simulink model "svpwm_inv_Motor_new_sent_split4"  (R2023a)
settings: Solver=daessc  StartTime=0.0  StopTime=0.62  MaxStep=2.5e-7  RelTol=1e-3
undefined symbols (not defined in the file): DiscIntNeverNeededParam
libraries: nesl_utility x37, fl_lib x34, ee_lib x21, spsMeanLib x7, simulink x6, mcbcontrolslib x4, slpidlib x4, sdl_lib x2, simulink_extras x1
(part 1 of 2)
settings Model: SimulationMode=rapid-accelerator  Creator=alexey  LastModifiedBy=alexey
settings SolverCC: ZeroCrossAlgorithm=Adaptive
settings OptimizationCC: ReuseModelBlockBuffer=off
settings DebuggingCC: IgnoredZcDiagnostic=none
settings GRTTargetCC: RTWCAPISignals=on  RTWCAPIParams=on

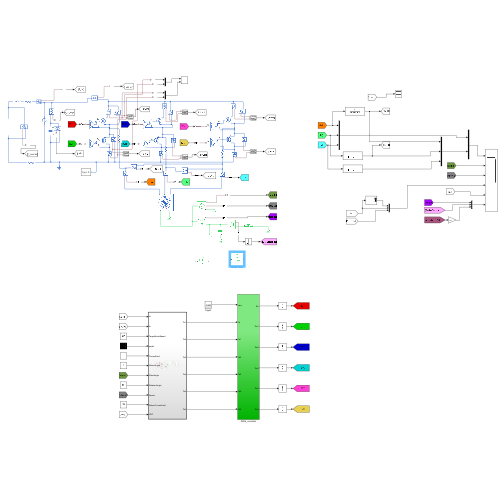
[thumbnail: Simulink's stored preview of the top-level diagram]
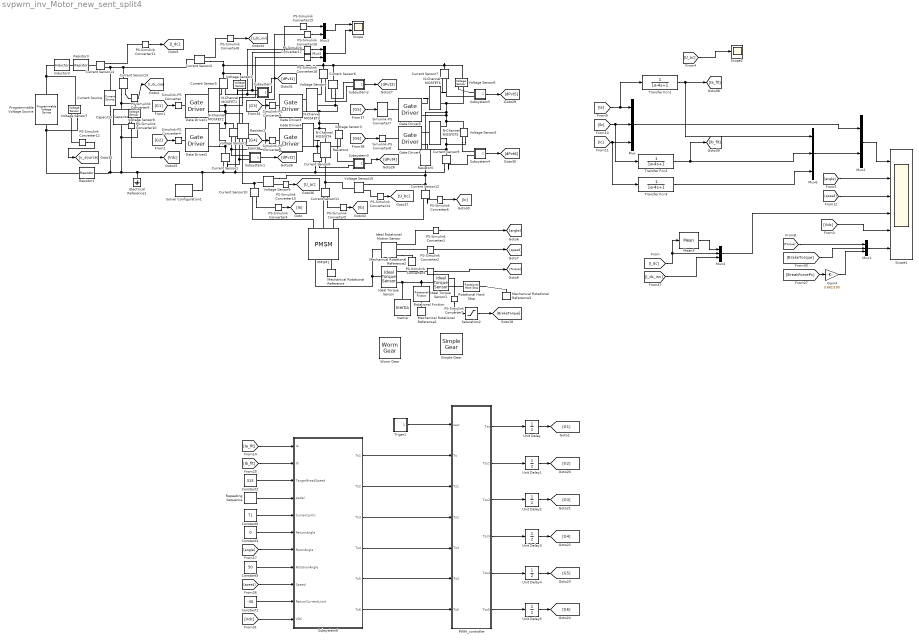
== system svpwm_inv_Motor_new_sent_split4 ==
  Capacitor : fl_lib/Electrical/Electrical Elements/Capacitor  c=270 uF  r=2 mOhm  g=0 1/Ohm  i_specify=off  i_priority=None  i=0 A  i_nominal_specify=off  i_nominal_unit=A  i_nominal_value=1  v_specify=on  v_priority=None  v=0 V  v_nominal_specify=off  v_nominal_unit=V  v_nominal_value=1  vc_specify=off  vc_priority=High  vc=0 V  vc_nominal_specify=off  vc_nominal_unit=V  vc_nominal_value=1
  Constant1 : Constant  Value=-30
  Constant2 : Constant  Value=315
  Constant4 : Constant  Value=0
  Constant5 : Constant  Value=50
  Constant6 : Constant  Value=71
  Current Sensor{1..2,5..14} (12 alike) : fl_lib/Electrical/Electrical Sensors/Current Sensor
  Current Source : ee_lib/Sources/Current Source  dc_current=0.25 A  ac_current=0 A  ac_shift=0 rad  ac_frequency=60 Hz  noise_mode=ee.enum.sources.noise.Disabled  PSD=0 A^2/Hz  sample_time=1e-3 s  repeatability=ee.enum.sources.repeatability.NotRepeatable  user_seed=0  auto_seed=3499211588  i_specify=off  i_priority=None  i=0 A  i_nominal_specify=off  i_nominal_unit=A  i_nominal_value=1  v_specify=off  v_priority=None  v=0 V  v_nominal_specify=off  v_nominal_unit=V  v_nominal_value=1
  Electrical Reference1 : fl_lib/Electrical/Electrical Elements/Electrical Reference
  Gain4 : Gain  Gain=3.682/100
  Gate Driver{1..6} (6 alike) : ee_lib/Semiconductors & Converters/Gate Driver  uHighValue=0.7  uLowValue=0.3  vHigh=12 V  vLow=0 V  tHigh=50 ns  tLow=50 ns  parameterization=1  rHigh=2 Ohm  rLow=2 Ohm  tRise=20 ns  tFall=20 ns  cLoad=10 nF  enable_faults=0  t_fault=1 s  fault_type=1  ZonTime_specify=off  ZonTime_priority=None  ZonTime=0 s  ZoffTime_specify=off  ZoffTime_priority=None  ZoffTime=0 s  uHigh=2.0 V  uLow=0.8 V
      settings: InternalSimscapePortConfiguration="{\"Bottom\":[],\"Left\":[{\"id\":\"u\",\"label\":\"u\",\"type\":\"input\"}],\"Right\":[{\"id\":\"G\",\"label\":\"G\",\"type\":\"foundation.electrical.electrical\"},{\"id\":\"S\",\"label\":\"S\",\"type\":\"foundation.electrical.electrical\"}],\"Top\":[]}"
  Ideal Rotational Motion Sensor : fl_lib/Mechanical/Mechanical Sensors/Ideal Rotational Motion Sensor  reference=foundation.enum.MeasurementReference.difference  acceleration_port=false  velocity_port=true  position_port=true  wrap_angle=false  offset=0 rad
  Ideal Torque Sensor : fl_lib/Mechanical/Mechanical Sensors/Ideal Torque Sensor
  Ideal Torque Sensor1 : fl_lib/Mechanical/Mechanical Sensors/Ideal Torque Sensor
  Inductor3 : ee_lib/Passive/Inductor  l=1 uH  enable_L_tol=0  L_tol=20  tol_distribution=1  nSigma=4  r=0 Ohm  g=1e-9 1/Ohm  enable_operating_limits=0  operating_limit_action=2  max_working_current=1 A  power_rating=1 W  enable_faults=ee.enum.enable.no  fault_action=simscape.enum.assert.action.none  lambdaPercent=50  k_faulted=0.9999  turnsShort=0  openCct=0  groundShort=0  groundShortG=0 1/Ohm  tau_fault=1e-3 s  fault_trigger=ee.enum.faults.faultTrigger.temporal  t_fault=1 s  max_permissible_voltage=100 V  n_fail_on_voltage=1  max_permissible_current=1 A  t_fail_on_current=1 s  i_L_specify=on  i_L_priority=High  i_L=0 A  i_L_nominal_specify=off  i_L_nominal_unit=A  i_L_nominal_value=1
  Inertia : fl_lib/Mechanical/Rotational Elements/Inertia  inertia=3e-5 kg*m^2  num_ports=foundation.enum.numPorts2.one  w_specify=off  w_priority=High  w=0 rad/s  w_nominal_specify=off  w_nominal_unit=rad/s  w_nominal_value=1  t_specify=off  t_priority=None  t=0 N*m  t_nominal_specify=off  t_nominal_unit=N*m  t_nominal_value=1
  Mean3 : spsMeanLib/Mean  Freq=10000  Vinit=0  Ts=0
  Mechanical Rotational Reference{,1..3} (4 alike) : fl_lib/Mechanical/Rotational Elements/Mechanical Rotational Reference
  Mux{,1,4,6} (4 alike) : Mux  Inputs=3
  Mux2 : Mux  Inputs=2
  Mux3 : Mux  Inputs=2
  Mux5 : Mux  Inputs=2
  N-Channel MOSFET{1..6} (6 alike) : ee_lib/Semiconductors & Converters/N-Channel MOSFET  paramTerminal=ee.enum.mosfet.numberOfTerminals.three  parameterization=ee.enum.mosfet.parameterization.datasheet  Beta=5.0 A/V^2  Rds=0.85 mOhm  Id=100 A  Vgs=10 V  Vth=2.6 V  Vth0=1.7 V  lam=0 1/V  gamma_vth=0.5 V^(1/2)  phib=0.5 V  Vth1=1.9071 V  Vbs1=-1 V  Vth2=2.066 V  Vbs2=-2 V  Tmeas=25 degC  Vgs_vec=[-.5, 2, 3, 4, 5] V  Vds_vec=[0, 2, 4, 8, 12, 16, 20] V  Vbs_vec=[0, -4, -6, -12] V  T_vec=[25, 125] degC  Vth_vec=[.4, 1.2, 1.4, 1.45] V  Vth_mat=[.4, .35; 1.2, 1.15; 1.4, 1.35; 1.45, 1.4] V  Ids_mat=[0, 0, 0, 0, 0, 0, 0; 0, .003, .0038, .0043, .0046, .0048, .0049; 0, .0055, .008, .009, .0095, .01, .0101; 0, .0115, .016, .018, .019, .0195, .02; 0, .0152, .0225, .0265, .028, .0295, .03] A  Ids_mat0=[0, 0, 0, 0, 0, 0, 0; 0, .003, .0038, .0043, .0046, .0048, .0049; 0, .0055, .008, .009, .0095, .01, .0101; 0, .0115, .016, .018, .019, .0195, .02; 0, .0152, .0225, .0265, .028, .0295, .03] A  Ids_mat_3D=zeros(5, 7, 2) A  Ids_mat_3D0=zeros(5, 7, 2) A  IV_table_symmetry=ee.enum.mosfet.symmetricNIV.no  RS=0.0001 Ohm  RD=0.0001 Ohm  RB=0.001 Ohm  C_param=ee.enum.mosfet.capacitanceParam.tabulatedciss  C_GS=270 pF  C_GD=80 pF  C_GB=0 pF  C_DS=0 pF  C_iss=350 pF  C_rss=80 pF  C_oss=0 pF  C_iss_vec=[19000, 17000, 16500, 16500, 16000, 16000, 16000, 16000, 16000] pF  C_rss_vec=[3100, 1700, 750, 280, 110, 90, 80, 80, 80] pF  C_oss_vec=[16000, 11000, 8000, 6500, 3000, 2800, 2650, 2600, 2400] pF  C_GS_vec=[270, 300, 290, 280, 295, 255] pF  C_GD_vec=[450, 400, 300, 190, 95, 55] pF  C_GB_vec=[270, 300, 290, 280, 295, 255] pF  C_Vgs_vec=0 V  C_DS_vec=[450, 410, 390, 230, 175, 115] pF  C_Vds_vec=[.1, 4, 12, 20, 28, 36, 44, 52, 60] V  V_GS_for_cap_data=0 V  charge_linearity_param=ee.enum.mosfet.cgdLinearity.constant  C_OX=200 pF  V_C_OX=-0.5 V  charge_linearity_param_vgb=ee.enum.mosfet.cgbLinearity.instantly  charge_linearity_param_with_vgb=ee.enum.mosfet.cgbLinearityWithSeparateCgb.instantly  Di_param=ee.enum.mosfet.diodeParam.tabulated  IsDiode=1e-12 A  Vbi=0.18 V  n=1  Cj0Diode=9000 pF  TT=50e-9 s  Tmeas_dio=25 degC  TableTypeNoT=ee.enum.mosfet.tableType.IfMat  TableType=ee.enum.diode.tableType.IfMat  IfVec=[1e-3, 1, 10, 100, 400, 1000] A  IfMat=[.07, .12, .19, 1.75, 4.24, 7.32, 11.2; .16, .3, .72, 2.14, 4.02, 6.35, 9.12] A  VfVecV=[.9, 1.15, 1.25, 1.5, 1.75, 2.17, 2.6, 2.85] V  VfMatV=[.9, 1.15, 1.25, 1.5, 1.75, 2.17, 2.6, 2.85; .58, .68, .75, 1.1, 1.38, 1.77, 2.27, 2.7] V  TjVec=[25, 125] degC  VfVec=[0.68, 0.69, 0.72, 0.82, 0.9, 1.1] V  IfVecV=[.1, .2, .5, 1, 2, 4, 7, 10] A  prmDatasheet=ee.enum.temperatureParameterization.none  prmEquCoeff=ee.enum.temperatureParameterization.none  dVth_dT=-6 mV/K  dVth0_dT=-6 mV/K  Rds_T2=0.037 Ohm  BEXDatasheet=-1.5  BEXEquCoeff=-1.5  etaisDatasheet=3  etaisEquCoeff=3  Tmeas2=125 degC  etaisTabulated=3  TdeviceDatasheet=25 degC  TdeviceEquCoeff=25 degC  TdeviceTabulated=25 degC  enable_faults=simscape.enum.onoff.off  fault_trigger=ee.enum.faults.faultTrigger.temporal  t_fault=inf s  max_permissible_Vgs=inf V  max_permissible_Vds=inf V  max_permissible_Vdb=inf V  max_permissible_Ids=inf A  t_fail_on_Ids=1 s  max_permissible_Idiode=inf A  t_fail_on_Idiode=1 s  max_permissible_dVdt=inf V/s  tau_fault=1e-3 s  fault_types=ee.enum.mosfet.faults.open  fault_types_4T=ee.enum.mosfet.faultsFourTerminals.open  RG_open=1e6 Ohm  RD_open=1000 Ohm  RS_open=1000 Ohm  RB_open=1000 Ohm  GDS_short=1000 1/Ohm  GDB_short=1000 1/Ohm  GSB_short=1000 1/Ohm  location_GOS=0  G_GOS=1000 1/Ohm  D_GOS=ee.enum.include.no  Is_GOS=0 A  Vbi_GOS=0.6 V  n_GOS=1  Cj0_GOS=0 pF  TT_GOS=50e-9 s  Beta_scale=100  dVth_faulted=0 V  lam_faulted=0 1/V  gamma_scale=100  dPhib_faulted=0 V  Vgs_vec_faulted=[-.5, 2, 3, 4, 5] V  Vds_vec_faulted=[0, 2, 4, 8, 12, 16, 20] V  Vbs_vec_faulted=[0, -4, -6, -12] V  Vth_vec_faulted=[.4, 1.2, 1.4, 1.45] V  Vth_mat_faulted=[.4, .35; 1.2, 1.15; 1.4, 1.35; 1.45, 1.4] V  Ids_mat_faulted=[0, 0, 0, 0, 0, 0, 0; 0, .003, .0038, .0043, .0046, .0048, .0049; 0, .0055, .008, .009, .0095, .01, .0101; 0, .0115, .016, .018, .019, .0195, .02; 0, .0152, .0225, .0265, .028, .0295, .03] A  Ids_mat0_faulted=[0, 0, 0, 0, 0, 0, 0; 0, .003, .0038, .0043, .0046, .0048, .0049; 0, .0055, .008, .009, .0095, .01, .0101; 0, .0115, .016, .018, .019, .0195, .02; 0, .0152, .0225, .0265, .028, .0295, .03] A  Ids_mat_3D_faulted=zeros(5, 7, 2) A  Ids_mat_3D0_faulted=zeros(5, 7, 2) A  RS_faulted=0.0001 Ohm  RD_faulted=0.01 Ohm  RB_faulted=0.001 Ohm  IsDiode_faulted=0 A  Vbi_faulted=0.6 V  n_faulted=1  Cj0Diode_scale=100  TT_faulted=50e-9 s  IfVec_faulted=[.07, .12, .19, 1.75, 4.24, 7.32, 11.2] A  IfMat_faulted=[.07, .12, .19, 1.75, 4.24, 7.32, 11.2; .16, .3, .72, 2.14, 4.02, 6.35, 9.12] A  VfVecV_faulted=[.9, 1.15, 1.25, 1.5, 1.75, 2.17, 2.6, 2.85] V  VfMatV_faulted=[.9, 1.15, 1.25, 1.5, 1.75, 2.17, 2.6, 2.85; .58, .68, .75, 1.1, 1.38, 1.77, 2.27, 2.7] V  VfVec_faulted=[.5, .7, .9, 1.3, 1.7, 2.1, 2.5] V  IfVecV_faulted=[.1, .2, .5, 1, 2, 4, 7, 10] A  C_GS_scale=100  C_GD_scale=100  C_GB_scale=100  C_DS_scale=100  C_OX_scale=100  V_C_OX_faulted=-0.5 V  C_iss_vec_faulted=[720, 700, 590, 470, 390, 310] pF  C_rss_vec_faulted=[450, 400, 300, 190, 95, 55] pF  C_oss_vec_faulted=[900, 810, 690, 420, 270, 170] pF  C_GS_vec_faulted=[270, 300, 290, 280, 295, 255] pF  C_GD_vec_faulted=[450, 400, 300, 190, 95, 55] pF  C_GB_vec_faulted=[270, 300, 290, 280, 295, 255] pF  C_Vgs_vec_faulted=0 V  C_DS_vec_faulted=[450, 410, 390, 230, 175, 115] pF  C_Vds_vec_faulted=[.1, .3, 1, 3, 10, 30] V  V_GS_for_cap_data_faulted=0 V  i_g_specify=off  i_g_priority=None  i_g=0 A  i_g_nominal_specify=off  i_g_nominal_unit=A  i_g_nominal_value=1  i_d_specify=on  i_d_priority=High  i_d=100 A  i_d_nominal_specify=off  i_d_nominal_unit=A  i_d_nominal_value=1  i_b_specify=off  i_b_priority=None  i_b=0 A  i_b_nominal_specify=off  i_b_nominal_unit=A  i_b_nominal_value=1  voltage_gs_specify=on  voltage_gs_priority=High  voltage_gs=0 V  voltage_gs_nominal_specify=off  voltage_gs_nominal_unit=V  voltage_gs_nominal_value=1  voltage_ds_specify=off  voltage_ds_priority=High  voltage_ds=12 V  voltage_ds_nominal_specify=off  voltage_ds_nominal_unit=V  voltage_ds_nominal_value=1  voltage_bs_specify=off  voltage_bs_priority=None  voltage_bs=0 V  voltage_bs_nominal_specify=off  voltage_bs_nominal_unit=V  voltage_bs_nominal_value=1  v_Cgs_specify=on  v_Cgs_priority=High  v_Cgs=0 V  v_Cgs_nominal_specify=off  v_Cgs_nominal_unit=V  v_Cgs_nominal_value=1  v_Cds_specify=on  v_Cds_priority=High  v_Cds=0 V  v_Cds_nominal_specify=off  v_Cds_nominal_unit=V  v_Cds_nominal_value=1  v_Cbs_specify=off  v_Cbs_priority=High  v_Cbs=0 V  v_Cbs_nominal_specify=off  v_Cbs_nominal_unit=V  v_Cbs_nominal_value=1  thermal_network_parameterization=ee.enum.thermalNetworkTopology.junctionCase  Rth=[0, 10] K/W  Rth_Cauer=[1, 3, 10] K/W  Rth_Foster=[4, 6] K/W  thermal_mass_parameterization=ee.enum.thermalNetwork.timeconstant  thermal_mass=[0, 1] J/K  thermal_mass_Cauer=[.1, .3, 1] J/K  thermal_mass_Foster=[1.5, 3] J/K  thermal_time_constant=[0, 10] s  thermal_time_constant_Cauer=[1, 3, 10] s  thermal_time_constant_Foster=[6, 18] s  thermal_mass_initial_temperatures=[25, 25] degC  thermal_mass_initial_temperatures_Cauer=[25, 25, 25] degC  Tvec_initial_Foster=[25, 25, 25, 25] degC  max_permissible_temperature=inf K  t_fail_on_temperature=1 s  betaref=18 A/V^2  Vfbref=-1.1 V  gamma=3.5 V^(1/2)  phib2ref=1 V  thesatref=0.4 1/V  alpha=0  Vp=5e-2 V  thesrref=0 1/V  m=8  Tref=25 degC  Rsref=2e-3 Ohm  Rdref=0.17 Ohm  Rgref=8.4 Ohm  Rbref=2e-3 Ohm  Cox=1500 pF  Cgso=100 pF  Cgdo=14 pF  Isref=5.2e-13 A  Cj0=480 pF  Tprm=1  etabet=1.3  Stvfb=5e-4 V/K  Stphib=-8.5e-4 V/K  etasat=1.04  etasr=0.65  etar=0.95  etais=3  Tsim=25 degC  Ig_specify=off  Ig_priority=None  Ig=0 A  Ig_nominal_specify=off  Ig_nominal_unit=A  Ig_nominal_value=1  Ids_specify=off  Ids_priority=None  Ids=0 A  Ids_nominal_specify=off  Ids_nominal_unit=A  Ids_nominal_value=1  Ib_specify=off  Ib_priority=None  Ib=0 A  Ib_nominal_specify=off  Ib_nominal_unit=A  Ib_nominal_value=1  V_gs_specify=off  V_gs_priority=None  V_gs=0 V  V_gs_nominal_specify=off  V_gs_nominal_unit=V  V_gs_nominal_value=1  V_ds_specify=off  V_ds_priority=None  V_ds=0 V  V_ds_nominal_specify=off  V_ds_nominal_unit=V  V_ds_nominal_value=1  V_bs_specify=off  V_bs_priority=None  V_bs=0 V  V_bs_nominal_specify=off  V_bs_nominal_unit=V  V_bs_nominal_value=1  QGoverCox_specify=off  QGoverCox_priority=None  QGoverCox=0 V  QGoverCox_nominal_specify=off  QGoverCox_nominal_unit=V  QGoverCox_nominal_value=1  QDoverCox_specify=off  QDoverCox_priority=None  QDoverCox=0 V  QDoverCox_nominal_specify=off  QDoverCox_nominal_unit=V  QDoverCox_nominal_value=1  QBoverCox_specify=off  QBoverCox_priority=None  QBoverCox=0 V  QBoverCox_nominal_specify=off  QBoverCox_nominal_unit=V  QBoverCox_nominal_value=1  T0=[25, 25] degC  T0_Cauer=[25, 25, 25] degC
  PMSM1 : ee_lib/Electromechanical/Permanent Magnet/PMSM  port_option=ee.enum.threePhasePort.expanded  winding_type=ee.enum.statorconnection.delta  machine_param=ee.enum.pmsm.parameterization.constant  nPolePairs=4  pmflux_param=ee.enum.pmflux.fluxlinkage  pm_flux_linkage=0.0163 Wb  torque_constant=0.074 N*m/A  back_emf_constant=0.06 V*s/rad  stator_param=ee.enum.statorparam.LdLqL0  Ld=119 uH  Lq=167 uH  idVec=[-200, 0, 200] A  iqVec=[-200, 0, 200] A  LdMatrix=0.0002 * ones(3, 3) H  LqMatrix=0.0002 * ones(3, 3) H  PmMatrix=0.1 * ones(3, 3) Wb  ktMatrix=0.18 * ones(3, 3) N*m/A  keMatrix=0.18 * ones(3, 3) V*s/rad  L0=1e-6 uH  Ls=0.0002 H  Lm=-0.00002 H  Ms=0.00002 H  Rs=0.1 Ohm  zero_sequence=ee.enum.park.zerosequence.include  axes_param=ee.enum.rotorangle.daxis  loss_param=ee.enum.ironloss.none  losses_oc=[0, 0, 0] W  losses_sc=[0, 0, 0] W  f_losses=60 Hz  Isc_losses=95 A  J=1e-8 kg*m^2  lam=0.00005 N*m*s/rad  i_d_specify=on  i_d_priority=None  i_d=0 A  i_d_nominal_specify=off  i_d_nominal_unit=A  i_d_nominal_value=1  i_q_specify=on  i_q_priority=None  i_q=0 A  i_q_nominal_specify=off  i_q_nominal_unit=A  i_q_nominal_value=1  torque_specify=on  torque_priority=None  torque=0 N*m  torque_nominal_specify=off  torque_nominal_unit=N*m  torque_nominal_value=1  angular_velocity_specify=off  angular_velocity_priority=High  angular_velocity=0 rpm  angular_velocity_nominal_specify=off  angular_velocity_nominal_unit=rpm  angular_velocity_nominal_value=1  angular_position_specify=off  angular_position_priority=High  angular_position=0 deg  angular_position_nominal_specify=off  angular_position_nominal_unit=deg  angular_position_nominal_value=1  alpha=3.93e-3 1/K  alpha_flux=-0.001 1/K  Tmeas=298.15 K  stator_thermal_mass=100 J/K  rotor_thermal_mass=200 J/K  Rm_percent_rotor=90  Rd_percent_rotor=30  temperatureA_specify=off  temperatureA_priority=High  temperatureA=25 degC  temperatureA_nominal_specify=off  temperatureA_nominal_unit=degC  temperatureA_nominal_value=1  temperatureB_specify=off  temperatureB_priority=High  temperatureB=25 degC  temperatureB_nominal_specify=off  temperatureB_nominal_unit=degC  temperatureB_nominal_value=1  temperatureC_specify=off  temperatureC_priority=High  temperatureC=25 degC  temperatureC_nominal_specify=off  temperatureC_nominal_unit=degC  temperatureC_nominal_value=1  temperatureR_specify=off  temperatureR_priority=High  temperatureR=25 degC  temperatureR_nominal_specify=off  temperatureR_nominal_unit=degC  temperatureR_nominal_value=1
      settings: InternalSimscapePortConfiguration="{\"Bottom\":[],\"Left\":[{\"id\":\"a\",\"label\":\"a\",\"type\":\"foundation.electrical.electrical\"},{\"id\":\"b\",\"label\":\"b\",\"type\":\"foundation.electrical.electrical\"},{\"id\":\"c\",\"label\":\"c\",\"type\":\"foundation.electrical.electrical\"}],\"Right\":[{\"id\":\"R\",\"label\":\"R\",\"type\":\"foundation.mechanical.rotational.rotational\"},{\"id\":\"C\",\"label\":\"C\",\"type\":\"foundation.mechanical.rotational.rotational\"}],\"Top\":[]}"
  PS-Simulink Converter{1..18} (18 alike) : nesl_utility/PS-Simulink Converter  PhysicalDomain=network_engine_domain  SubClassName=ps_output  LeftPortType=input  RightPortType=output  PseudoPeriodic=off  Frequencies=[]  VectorFormat=inherit  Unit=inherit  AffineConversion=off
  PWM_controller : Subsystem
  Programmable Voltage Source : ee_lib/Sources/Programmable Voltage Source  magnitude_type=ee.enum.timechanging.constant  ac_magnitude=0 V  magn_ramp=1 V/s  magn_step=1 V  magn_modu_magn=1 V  magn_modu_freq=1 Hz  magn_t1=1 s  magn_t2=2 s  frequency_type=ee.enum.timechanging.constant  ac_frequency=60 Hz  freq_ramp=1 Hz/s  freq_step=1 Hz  freq_modu_magn=1 Hz  freq_modu_freq=1 Hz  freq_t1=1 s  freq_t2=2 s  phase_type=ee.enum.timechanging.constant  ac_shift=0 deg  phase_ramp=1 deg/s  phase_step=1 deg  phase_modu_magn=1 deg  phase_modu_freq=1 Hz  phase_t1=1 s  phase_t2=2 s  dc_type=ee.enum.timechanging.ramp  dc_voltage=0 V  dc_ramp=24000 V/s  dc_step=24 V  dc_modu_magn=1 V  dc_modu_freq=1 Hz  dc_t1=0 s  dc_t2=100e-5 s  harmonic_option=0  harmonic_orders=[5, 7, 11, 13]  harmonic_ratios=[.1, .1, .1, .1]  harmonic_shifts=[0, 0, 0, 0] deg  harmonic_t1=-inf s  harmonic_t2=inf s  noise_mode=0  PSD=0 V^2/Hz  repeatability=1  auto_seed=0  user_seed=0  sample_time=1e-3 s  i_specify=off  i_priority=None  i=0 A  i_nominal_specify=off  i_nominal_unit=A  i_nominal_value=1  v_specify=on  v_priority=High  v=0 V  v_nominal_specify=off  v_nominal_unit=V  v_nominal_value=1
      settings: InternalSimscapePortConfiguration="{\"Bottom\":[],\"Left\":[{\"id\":\"p\",\"label\":\"+\",\"type\":\"foundation.electrical.electrical\"}],\"Right\":[{\"id\":\"n\",\"label\":\"-\",\"type\":\"foundation.electrical.electrical\"}],\"Top\":[]}"
  Repeating Sequence : simulink/Sources/Repeating Sequence  rep_seq_t=[0 0.4 0.6 0.61 1 1.4 1.6 1.61 2 2.05 2.08 2.081 2.5 2.501 2.8 2.9 3]  rep_seq_y="[0 100 100 0 0  15 15 0 0 55 95 0 0 100 100 70 0]"
  Resistor1 : ee_lib/Passive/Resistor  R=40 mOhm  enable_R_tol=0  R_tol=5  tol_distribution=1  nSigma=4  enable_operating_limits=0  operating_limit_action=2  power_rating=1 W  max_working_voltage=100 V  enable_faults=ee.enum.enable.no  fault_action=simscape.enum.assert.action.none  R_faulted=inf Ohm  fault_trigger=ee.enum.faults.faultTrigger.temporal  t_fault=1 s  max_permissible_current=1 A  t_fail_on_current=1 s  noise_mode=0  Tdevice=25 degC  sample_time=1e-3 s  repeatability=1  user_seed=0  auto_seed=3890346746  power_derating_T1=70 degC  power_derating_T2=155 degC  operating_temperature_range_vec=[-50, 150] degC  alpha=3.93e-3 1/K  Tmeas=25 degC  thermal_mass=100 J/K  temperature_specify=off  temperature_priority=High  temperature=298.15 K  temperature_nominal_specify=off  temperature_nominal_unit=K  temperature_nominal_value=1
  Resistor2 : ee_lib/Passive/Resistor  R=0.1 mOhm  enable_R_tol=0  R_tol=5  tol_distribution=1  nSigma=4  enable_operating_limits=0  operating_limit_action=2  power_rating=1 W  max_working_voltage=100 V  enable_faults=ee.enum.enable.no  fault_action=simscape.enum.assert.action.none  R_faulted=inf Ohm  fault_trigger=ee.enum.faults.faultTrigger.temporal  t_fault=1 s  max_permissible_current=1 A  t_fail_on_current=1 s  noise_mode=0  Tdevice=25 degC  sample_time=1e-3 s  repeatability=1  user_seed=0  auto_seed=545404223  power_derating_T1=70 degC  power_derating_T2=155 degC  operating_temperature_range_vec=[-50, 150] degC  alpha=3.93e-3 1/K  Tmeas=25 degC  thermal_mass=100 J/K  temperature_specify=off  temperature_priority=High  temperature=298.15 K  temperature_nominal_specify=off  temperature_nominal_unit=K  temperature_nominal_value=1
  Resistor3 : ee_lib/Passive/Resistor  R=40 mOhm  enable_R_tol=0  R_tol=5  tol_distribution=1  nSigma=4  enable_operating_limits=0  operating_limit_action=2  power_rating=1 W  max_working_voltage=100 V  enable_faults=ee.enum.enable.no  fault_action=simscape.enum.assert.action.none  R_faulted=inf Ohm  fault_trigger=ee.enum.faults.faultTrigger.temporal  t_fault=1 s  max_permissible_current=1 A  t_fail_on_current=1 s  noise_mode=0  Tdevice=25 degC  sample_time=1e-3 s  repeatability=1  user_seed=0  auto_seed=545404223  power_derating_T1=70 degC  power_derating_T2=155 degC  operating_temperature_range_vec=[-50, 150] degC  alpha=3.93e-3 1/K  Tmeas=25 degC  thermal_mass=100 J/K  temperature_specify=off  temperature_priority=High  temperature=298.15 K  temperature_nominal_specify=off  temperature_nominal_unit=K  temperature_nominal_value=1
  Resistor4 : ee_lib/Passive/Resistor  R=0.1 mOhm  enable_R_tol=0  R_tol=5  tol_distribution=1  nSigma=4  enable_operating_limits=0  operating_limit_action=2  power_rating=1 W  max_working_voltage=100 V  enable_faults=ee.enum.enable.no  fault_action=simscape.enum.assert.action.none  R_faulted=inf Ohm  fault_trigger=ee.enum.faults.faultTrigger.temporal  t_fault=1 s  max_permissible_current=1 A  t_fail_on_current=1 s  noise_mode=0  Tdevice=25 degC  sample_time=1e-3 s  repeatability=1  user_seed=0  auto_seed=2715962282  power_derating_T1=70 degC  power_derating_T2=155 degC  operating_temperature_range_vec=[-50, 150] degC  alpha=3.93e-3 1/K  Tmeas=25 degC  thermal_mass=100 J/K  temperature_specify=off  temperature_priority=High  temperature=298.15 K  temperature_nominal_specify=off  temperature_nominal_unit=K  temperature_nominal_value=1
  Resistor5 : ee_lib/Passive/Resistor  R=0.1 mOhm  enable_R_tol=0  R_tol=5  tol_distribution=1  nSigma=4  enable_operating_limits=0  operating_limit_action=2  power_rating=1 W  max_working_voltage=100 V  enable_faults=ee.enum.enable.no  fault_action=simscape.enum.assert.action.none  R_faulted=inf Ohm  fault_trigger=ee.enum.faults.faultTrigger.temporal  t_fault=1 s  max_permissible_current=1 A  t_fail_on_current=1 s  noise_mode=0  Tdevice=25 degC  sample_time=1e-3 s  repeatability=1  user_seed=0  auto_seed=418932850  power_derating_T1=70 degC  power_derating_T2=155 degC  operating_temperature_range_vec=[-50, 150] degC  alpha=3.93e-3 1/K  Tmeas=25 degC  thermal_mass=100 J/K  temperature_specify=off  temperature_priority=High  temperature=298.15 K  temperature_nominal_specify=off  temperature_nominal_unit=K  temperature_nominal_value=1
  Rotational Friction : fl_lib/Mechanical/Rotational Elements/Rotational Friction  brkwy_trq=0.31 N*m  brkwy_vel=0.01 rad/s  Col_trq=0.3 N*m  visc_coef=0.1189 N*m*s/rad  w_specify=off  w_priority=None  w=0 rad/s  w_nominal_specify=off  w_nominal_unit=rad/s  w_nominal_value=1  t_specify=off  t_priority=None  t=0 N*m  t_nominal_specify=off  t_nominal_unit=N*m  t_nominal_value=1
  Rotational Hard Stop : fl_lib/Mechanical/Rotational Elements/Rotational Hard Stop  upper_bnd=14.8*pi/14.8 rad  lower_bnd=(-2*pi) rad  model=simscape.enum.hardstop.fulldamped  stiff_up=1e6 N*m/rad  stiff_low=1e6 N*m/rad  D_up=1500 N*m*s/rad  D_low=1500 N*m*s/rad  transition=0.001 rad  coeff_rest=0.7  w_tol=0.1 rad/s  trq_tol=0.001 N*m  phi_specify=off  phi_priority=High  phi=0 rad  phi_nominal_specify=off  phi_nominal_unit=rad  phi_nominal_value=1  w_specify=off  w_priority=None  w=0 rad/s  w_nominal_specify=off  w_nominal_unit=rad/s  w_nominal_value=1  t_specify=off  t_priority=None  t=0 N*m  t_nominal_specify=off  t_nominal_unit=N*m  t_nominal_value=1  M_specify=off  M_priority=None  M=0
  Saturation2 : Saturate  UpperLimit=5  LowerLimit=0
  Scope : Scope  NumInputPorts=2
  Scope1 : Scope  NumInputPorts=6
  Scope2 : Scope
  Simple Gear : sdl_lib/Gears/Simple Gear  ratio=2  rotation_direction=sdl.enum.shaftOutputDirection.opposite  friction_model=sdl.enum.gear_efficiencies_load.loadDependent  T_noload=0.1 N*m  T_nom=5 N*m  efficiency_nom=0.8  efficiency=0.8  temperature_TLU=[280, 300, 320] K  load_TLU=[1, 5, 10] N*m  efficiency_TLU=[.95, .9, .85]  efficiency_TLU2=[.85, .8, .75; .95, .9, .85; .85, .8, .7]  w_thr=0.01 rad/s  pwr_thr=0.001 W  enable_backlash=true  hardstop_model=simscape.enum.hardstop.smooth  backlash_distance=1e-3 mm  r_base=0.1 m  transition=1e-4 mm  backlash_stiffness=1e6 N/m  backlash_damping=1e3 N*s/m  coeff_rest=0.7  v_tol=0.001 m/s  f_tol=0.001 N  mu_visc=[0, 0] N*m*s/rad  enable_faults=simscape.enum.onoff.off  efficiency_fault=0.05  external_fault=simscape.enum.onoff.off  temporal_fault=simscape.enum.onoff.off  fault_time=5 s  fault_angles=pi / 12 rad  report_fault=simscape.enum.assert.action.none  thermal_mass=50 J/K  temperature_specify=off  temperature_priority=High  temperature=300 K  temperature_nominal_specify=off  temperature_nominal_unit=K  temperature_nominal_value=1  x_backlash_specify=off  x_backlash_priority=None  x_backlash=0 mm  x_backlash_nominal_specify=off  x_backlash_nominal_unit=mm  x_backlash_nominal_value=1  f_hardstop_specify=off  f_hardstop_priority=None  f_hardstop=0 N  f_hardstop_nominal_specify=off  f_hardstop_nominal_unit=N  f_hardstop_nominal_value=1  v_backlash_specify=off  v_backlash_priority=None  v_backlash=0 m/s  v_backlash_nominal_specify=off  v_backlash_nominal_unit=m/s  v_backlash_nominal_value=1
  Simulink-PS Converter{,4..8} (6 alike) : nesl_utility/Simulink-PS Converter  PhysicalDomain=network_engine_domain  SubClassName=ps_input  LeftPortType=input  RightPortType=output  PseudoPeriodic=off  Frequencies=[]  NoiseDistribution=none  NoiseParameters=[]  Unit=1  AffineConversion=off  FilteringAndDerivatives=provide  SimscapeFilterOrder=1  InputFilterTimeConstant=0.001  UdotUserProvided=0
  Solver Configuration1 : nesl_utility/Solver Configuration  PhysicalDomain=network_engine_domain  SubClassName=solver  LeftPortType=input  RightPortType=generic  Tones=[]  Harmonics=[]  SimulateNoise=off  Profile=off  UseLocalSampling=off  EnableSwitchedLinearOptims=on  FrequencyDomain=off  UseCCode=off  RelTol=0.001  AbsTol=0.001  MinStep=1e-09  ToWorkspace=off  RevertToSquareIcSolve=off  NumHomotopyIterations=100  PhasorMode=off  PhasorModeNumHarmonics=1  ConsistencySolver=NEWTON_XTOL_AFTER_FTOL  IndexReductionMethod=DerivativeReplacement  DoDC=off  ResidualTolerance=1e-09  ConsistencyTolSource=GLOBAL  ConsistencyAbsTol=0.001  ConsistencyRelTol=0.001  ConsistencyTolFactor=0.001  UseLocalSolver=off  LocalSolverChoice=NE_BACKWARD_EULER_ADVANCER  ResolveIndetEquations=on  FunctionEvalNumThread=1  LocalSolverSampleTime=0.001  DoFixedCost=off  MaxNonlinIter=3  MaxModeIter=2  ComputeImpulses=off  ImpulseIterations=2  LinearAlgebra=auto  LinearAlgebraNumThread=0  EquationFormulation=NE_TIME_EF  DelaysMemoryBudget=1024  AutomaticFiltering=on  FilteringTimeConstant=0.001  PartitionStorageMethod=AS_NEEDED  PartitionMemoryBudget=1024  PartitionMethod=ROBUST
  Subsystem : Subsystem
  Subsystem1 : Subsystem
  Subsystem2 : Subsystem
  Subsystem3 : Subsystem
  Subsystem4 : Subsystem
  Subsystem5 : Subsystem
  Subsystem6 : Subsystem  TreatAsAtomicUnit=on  SystemSampleTime=80e-6
  Transfer Fcn1 : TransferFcn  Denominator=[1e-4 1]
  Transfer Fcn2 : TransferFcn  Denominator=[1e-4 1]
  Transfer Fcn3 : TransferFcn  Denominator=[1e-4 1]
  Triger1 : Subsystem
  Unit Delay{,1..5} (6 alike) : UnitDelay  SampleTime=1e-6  HasFrameUpgradeWarning=on
  Voltage Sensor{1..10} (10 alike) : fl_lib/Electrical/Electrical Sensors/Voltage Sensor
  Worm Gear : sdl_lib/Gears/Worm Gear  ratio=25  thread_type=sdl.enum.handedness.right  friction_model=sdl.enum.gear_friction.constant  friction_parameterization=sdl.enum.efficiency_geometry.geometry  pr_ang=17.5 deg  lead_ang=20 deg  fr_coeff=0.08  eff_wg=0.74  eff_gw=0.65  temperature_TLU=[280, 300, 320] K  efficiency_wg_TLU=[.75, .65, .6]  efficiency_gw_TLU=[.5, .45, .4]  pwr_thr=0.001 W  mu_visc=[0, 0] N*m*s/rad  thermal_mass=50 J/K  temperature_specify=off  temperature_priority=High  temperature=300 K  temperature_nominal_specify=off  temperature_nominal_unit=K  temperature_nominal_value=1
      settings: InternalSimscapePortConfiguration="{\"Bottom\":[],\"Left\":[{\"id\":\"W\",\"label\":\"W\",\"type\":\"foundation.mechanical.rotational.rotational\"}],\"Right\":[{\"id\":\"G\",\"label\":\"G\",\"type\":\"foundation.mechanical.rotational.rotational\"}],\"Top\":[]}"
  wires:
  [Torque] -> Mux1/1
  PS-Simulink Converter1/1 -> [angle]
  PS-Simulink Converter2/1 -> [speed]
  PS-Simulink Converter3/1 -> [Torque]
  Mux/1 -> Mux2/1
  [Ia] -> Transfer Fcn1/1, Mux/1
  [Ib] -> Transfer Fcn2/1, Mux/2
  [Ic] -> Mux/3, Transfer Fcn3/1
  [angle] -> Scope1/2
  [speed] -> Scope1/3
  Mux1/1 -> Scope1/6
  Gain4/1 -> Mux1/3
  PS-Simulink Converter7/1 -> Saturation2/1
  Saturation2/1 -> [BrakeTorque]
  [BrakeTorque] -> Mux1/2
  PWM_controller/3(Tss2) -> Unit Delay2/1
  PWM_controller/2(Tss1) -> Unit Delay1/1
  PWM_controller/6(Tss5) -> Unit Delay5/1
  Subsystem6/1(Ts1) -> PWM_controller/2(Ts)
  PWM_controller/1(Tss) -> Unit Delay/1
  PWM_controller/5(Tss4) -> Unit Delay4/1
  Triger1/1(SAW) -> PWM_controller/1(saw)
  PWM_controller/4(Tss3) -> Unit Delay3/1
  PS-Simulink Converter9/1 -> [I_dc_cap]
  PS-Simulink Converter5/1 -> [Ib]
  Subsystem5/1(Power) -> [dPvt5]
  Subsystem2/1(Power) -> [dPvt3]
  Subsystem4/1(Power) -> [dPvt6]
  Subsystem1/1(Power) -> [dPvt2]
  PS-Simulink Converter6/1 -> [Ic]
  Subsystem/1(Power) -> [dPvt1]
  PS-Simulink Converter10/1 -> [Vdc]
  [G1] -> Simulink-PS Converter/1
  Subsystem3/1(Power) -> [dPvt4]
  [G4] -> Simulink-PS Converter6/1
  [G5] -> Simulink-PS Converter7/1
  PS-Simulink Converter4/1 -> [Ia]
  [G6] -> Simulink-PS Converter8/1
  PS-Simulink Converter11/1 -> [I_dc]
  [G3] -> Simulink-PS Converter5/1
  [G2] -> Simulink-PS Converter4/1
  PS-Simulink Converter8/1 -> [I_dc_inv]
  PS-Simulink Converter12/1 -> [v_source]
  PS-Simulink Converter13/1 -> [U_ac]
  PS-Simulink Converter14/1 -> [U_bc]
  [I_dc_inv] -> Mux4/3
  [I_dc] -> Mean3/1, Mux4/2
  Mean3/1 -> Mux4/1
  Mux4/1 -> Scope1/4
  [BreakForcePc] -> Gain4/1
  Mux2/1 -> Scope1/1
  PS-Simulink Converter15/1 -> Mux3/1
  Mux3/1 -> Scope/1
  PS-Simulink Converter16/1 -> Mux3/2
  PS-Simulink Converter18/1 -> Mux5/2
  PS-Simulink Converter17/1 -> Mux5/1
  Mux5/1 -> Scope/2
  Mux6/1 -> Mux2/2
  Transfer Fcn1/1 -> [Ia_flt], Mux6/1
  Transfer Fcn2/1 -> Mux6/2, [Ib_flt]
  Transfer Fcn3/1 -> Mux6/3
  [Ia_flt] -> Subsystem6/1(Ia)
  [Ib_flt] -> Subsystem6/2(Ib)
  Constant2/1 -> Subsystem6/3(TargerBreakSpeed)
  Repeating Sequence/1 -> Subsystem6/4(pedal)
  Constant6/1 -> Subsystem6/5(CurrentLimit)
  Constant4/1 -> Subsystem6/6(ReturnAngle)
  [angle] -> Subsystem6/7(RotorAngle)
  Constant5/1 -> Subsystem6/8(RotationAngle)
  [speed] -> Subsystem6/9(Speed)
  Constant1/1 -> Subsystem6/10(ReturnCurrentLimit)
  [Vdc] -> Subsystem6/11(VDC)
  Subsystem6/2(Ts2) -> PWM_controller/3(Ts1)
  Subsystem6/3(Ts3) -> PWM_controller/4(Ts2)
  Subsystem6/4(Ts4) -> PWM_controller/5(Ts3)
  Subsystem6/5(Ts5) -> PWM_controller/6(Ts4)
  Subsystem6/6(Ts6) -> PWM_controller/7(Ts5)
  Unit Delay/1 -> [G1]
  Unit Delay1/1 -> [G2]
  Unit Delay2/1 -> [G3]
  Unit Delay3/1 -> [G4]
  Unit Delay4/1 -> [G5]
  Unit Delay5/1 -> [G6]
  [Vdc] -> Scope1/5
  [U_ac] -> Scope2/1
  connections:
  Mechanical Rotational Reference/LConn1 -- PMSM1/RConn2
  Ideal Torque Sensor/LConn1 -- PMSM1/RConn1 -- Ideal Rotational Motion Sensor/LConn1
  Ideal Rotational Motion Sensor/RConn1 -- Mechanical Rotational Reference2/LConn1
  PS-Simulink Converter1/LConn1 -- Ideal Rotational Motion Sensor/RConn3
  PS-Simulink Converter2/LConn1 -- Ideal Rotational Motion Sensor/RConn2
  PS-Simulink Converter3/LConn1 -- Ideal Torque Sensor/RConn2
  Inertia/LConn1 -- Rotational Friction/LConn1 -- Ideal Torque Sensor1/LConn1 -- Ideal Torque Sensor/RConn1
  Rotational Friction/RConn1 -- Mechanical Rotational Reference1/LConn1
  Ideal Torque Sensor1/RConn1 -- Rotational Hard Stop/LConn1
  Ideal Torque Sensor1/RConn2 -- PS-Simulink Converter7/LConn1
  Voltage Sensor2/LConn1 -- Current Sensor5/LConn1 -- Current Sensor2/RConn2 -- Current Sensor6/LConn1 -- Current Sensor7/LConn1 -- Voltage Sensor6/LConn1 -- Voltage Sensor4/LConn1
  N-Channel MOSFET5/RConn2 -- Voltage Sensor5/RConn2 -- Current Sensor9/LConn1 -- Gate Driver6/RConn2
  Current Sensor8/RConn2 -- Current Sensor9/RConn2 -- Voltage Sensor1/RConn2 -- Current Sensor1/RConn2 -- Solver Configuration1/RConn1 -- Electrical Reference1/LConn1 -- Voltage Sensor8/RConn2 -- Capacitor/RConn1 -- Resistor1/LConn1 -- Current Source/LConn1
  Voltage Sensor1/LConn1 -- Gate Driver1/RConn2 -- N-Channel MOSFET1/RConn2 -- Voltage Sensor2/RConn2 -- Resistor2/LConn1 -- N-Channel MOSFET2/RConn1
  N-Channel MOSFET3/RConn2 -- Voltage Sensor3/LConn1 -- Resistor4/LConn1 -- N-Channel MOSFET4/RConn1 -- Gate Driver3/RConn2 -- Voltage Sensor4/RConn2
  Capacitor/LConn1 -- Current Sensor13/RConn2 -- Voltage Sensor8/LConn1
  Gate Driver4/RConn2 -- Current Sensor8/LConn1 -- N-Channel MOSFET4/RConn2 -- Voltage Sensor3/RConn2
  Current Sensor1/LConn1 -- Gate Driver2/RConn2 -- N-Channel MOSFET2/RConn2
  Voltage Sensor10/RConn2 -- Current Sensor12/LConn1 -- Resistor5/RConn1 -- Voltage Sensor9/RConn2
  Resistor3/RConn1 -- Inductor3/RConn1
  Subsystem3/LConn1 -- Voltage Sensor3/RConn1
  Voltage Sensor2/RConn1 -- PS-Simulink Converter15/LConn1 -- Subsystem/LConn1
  Gate Driver6/LConn1 -- Simulink-PS Converter8/RConn1
  Gate Driver1/RConn1 -- N-Channel MOSFET1/LConn1
  Current Sensor6/RConn2 -- N-Channel MOSFET3/RConn1
  Current Sensor9/RConn1 -- Subsystem4/LConn2
  Inductor3/LConn1 -- Voltage Sensor7/LConn1 -- Programmable Voltage Source/LConn1
  Gate Driver3/RConn1 -- N-Channel MOSFET3/LConn1
  Voltage Sensor5/RConn1 -- Subsystem4/LConn1
  Current Sensor13/RConn1 -- PS-Simulink Converter9/LConn1
  Current Sensor11/RConn1 -- PS-Simulink Converter5/LConn1
  Gate Driver2/LConn1 -- Simulink-PS Converter4/RConn1
  PMSM1/LConn1 -- Current Sensor10/RConn2
  Current Sensor14/LConn1 -- Resistor3/LConn1
  N-Channel MOSFET2/LConn1 -- Gate Driver2/RConn1
  PMSM1/LConn2 -- Current Sensor11/RConn2
  Current Sensor1/RConn1 -- PS-Simulink Converter18/LConn1 -- Subsystem1/LConn2
  N-Channel MOSFET6/LConn1 -- Gate Driver5/RConn1
  PMSM1/LConn3 -- Current Sensor12/RConn2
  Subsystem2/LConn2 -- Current Sensor6/RConn1
  Subsystem5/LConn1 -- Voltage Sensor6/RConn1
  Voltage Sensor8/RConn1 -- PS-Simulink Converter10/LConn1
  Subsystem5/LConn2 -- Current Sensor7/RConn1
  Simulink-PS Converter7/RConn1 -- Gate Driver5/LConn1
  Subsystem2/LConn1 -- Voltage Sensor4/RConn1
  Current Sensor5/RConn1 -- PS-Simulink Converter17/LConn1 -- Subsystem/LConn2
  Current Sensor12/RConn1 -- PS-Simulink Converter6/LConn1
  Simulink-PS Converter5/RConn1 -- Gate Driver3/LConn1
  N-Channel MOSFET5/LConn1 -- Gate Driver6/RConn1
  N-Channel MOSFET6/RConn1 -- Current Sensor7/RConn2
  Voltage Sensor1/RConn1 -- PS-Simulink Converter16/LConn1 -- Subsystem1/LConn1
  Gate Driver4/LConn1 -- Simulink-PS Converter6/RConn1
  Current Sensor8/RConn1 -- Subsystem3/LConn2
  Simulink-PS Converter/RConn1 -- Gate Driver1/LConn1
  Current Sensor10/RConn1 -- PS-Simulink Converter4/LConn1
  Current Sensor14/RConn1 -- PS-Simulink Converter11/LConn1
  N-Channel MOSFET4/LConn1 -- Gate Driver4/RConn1
  Current Sensor5/RConn2 -- N-Channel MOSFET1/RConn1
  Rotational Hard Stop/RConn1 -- Mechanical Rotational Reference3/LConn1
  PS-Simulink Converter8/LConn1 -- Current Sensor2/RConn1
  PS-Simulink Converter12/LConn1 -- Voltage Sensor7/RConn1
  PS-Simulink Converter14/LConn1 -- Voltage Sensor10/RConn1
  PS-Simulink Converter13/LConn1 -- Voltage Sensor9/RConn1
  Current Sensor14/RConn2 -- Current Sensor2/LConn1 -- Current Sensor13/LConn1 -- Current Source/RConn1
  Voltage Sensor7/RConn2 -- Resistor1/RConn1 -- Programmable Voltage Source/RConn1
  Resistor2/RConn1 -- Voltage Sensor9/LConn1 -- Current Sensor10/LConn1
  Current Sensor11/LConn1 -- Resistor4/RConn1 -- Voltage Sensor10/LConn1
  Voltage Sensor6/RConn2 -- N-Channel MOSFET5/RConn1 -- Voltage Sensor5/LConn1 -- Gate Driver5/RConn2 -- Resistor5/LConn1 -- N-Channel MOSFET6/RConn2

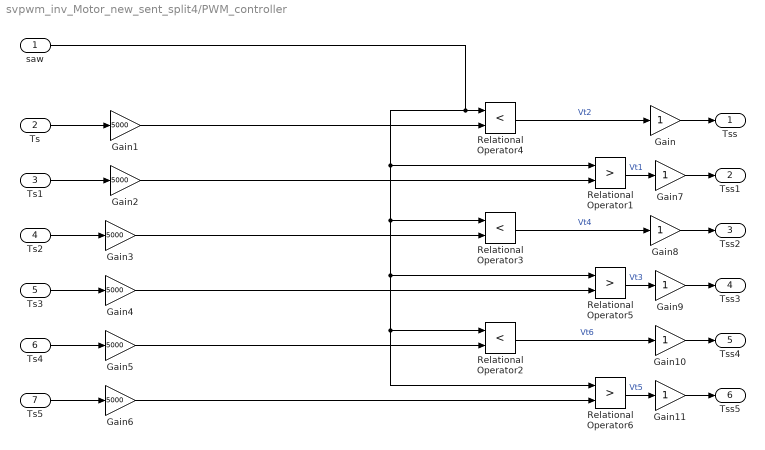
== system svpwm_inv_Motor_new_sent_split4/PWM_controller ==
  saw : Inport
  Ts : Inport  Port=2
  Ts1 : Inport  Port=3
  Ts2 : Inport  Port=4
  Ts3 : Inport  Port=5
  Ts4 : Inport  Port=6
  Ts5 : Inport  Port=7
  Gain{,7..11} (6 alike) : Gain  OutDataTypeStr=double
  Gain{1..6} (6 alike) : Gain  Gain=5000
  Relational Operator1 : RelationalOperator  Operator=>  OutDataTypeStr=boolean  InputSameDT=off
  Relational Operator2 : RelationalOperator  Operator=<  OutDataTypeStr=boolean  InputSameDT=off
  Relational Operator3 : RelationalOperator  Operator=<  OutDataTypeStr=boolean  InputSameDT=off
  Relational Operator4 : RelationalOperator  Operator=<  OutDataTypeStr=boolean  InputSameDT=off
  Relational Operator5 : RelationalOperator  Operator=>  OutDataTypeStr=boolean  InputSameDT=off
  Relational Operator6 : RelationalOperator  Operator=>  OutDataTypeStr=boolean  InputSameDT=off
  Tss : Outport  VectorParamsAs1DForOutWhenUnconnected=off
  Tss1 : Outport  Port=2  VectorParamsAs1DForOutWhenUnconnected=off
  Tss2 : Outport  Port=3  VectorParamsAs1DForOutWhenUnconnected=off
  Tss3 : Outport  Port=4  VectorParamsAs1DForOutWhenUnconnected=off
  Tss4 : Outport  Port=5  VectorParamsAs1DForOutWhenUnconnected=off
  Tss5 : Outport  Port=6  VectorParamsAs1DForOutWhenUnconnected=off
  wires:
  Relational Operator4/1 -> Gain/1  "Vt2"
  Gain3/1 -> Relational Operator3/2
  Gain5/1 -> Relational Operator2/2
  Relational Operator3/1 -> Gain8/1  "Vt4"
  Relational Operator2/1 -> Gain10/1  "Vt6"
  Ts/1 -> Gain1/1
  saw/1 -> Relational Operator1/1, Relational Operator3/1, Relational Operator5/1, Relational Operator2/1, Relational Operator6/1, Relational Operator4/1
  Relational Operator1/1 -> Gain7/1  "Vt1"
  Relational Operator5/1 -> Gain9/1  "Vt3"
  Relational Operator6/1 -> Gain11/1  "Vt5"
  Gain2/1 -> Relational Operator1/2
  Gain4/1 -> Relational Operator5/2
  Gain6/1 -> Relational Operator6/2
  Gain1/1 -> Relational Operator4/2
  Ts1/1 -> Gain2/1
  Ts2/1 -> Gain3/1
  Ts3/1 -> Gain4/1
  Ts4/1 -> Gain5/1
  Ts5/1 -> Gain6/1
  Gain/1 -> Tss/1
  Gain7/1 -> Tss1/1
  Gain8/1 -> Tss2/1
  Gain9/1 -> Tss3/1
  Gain10/1 -> Tss4/1
  Gain11/1 -> Tss5/1

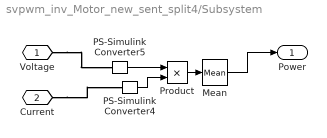
== system svpwm_inv_Motor_new_sent_split4/Subsystem ==
  Mean : spsMeanLib/Mean  Freq=5000  Vinit=0  Ts=0
  PS-Simulink Converter4 : nesl_utility/PS-Simulink Converter  PhysicalDomain=network_engine_domain  SubClassName=ps_output  LeftPortType=input  RightPortType=output  PseudoPeriodic=off  Frequencies=[]  VectorFormat=inherit  Unit=inherit  AffineConversion=off
  PS-Simulink Converter5 : nesl_utility/PS-Simulink Converter  PhysicalDomain=network_engine_domain  SubClassName=ps_output  LeftPortType=input  RightPortType=output  PseudoPeriodic=off  Frequencies=[]  VectorFormat=inherit  Unit=inherit  AffineConversion=off
  Product : Product
  Voltage : PMIOPort  Side=Left
  Current : PMIOPort  Port=2  Side=Left
  Power : Outport
  wires:
  Product/1 -> Mean/1
  PS-Simulink Converter5/1 -> Product/1
  PS-Simulink Converter4/1 -> Product/2
  Mean/1 -> Power/1
  connections:
  Current/RConn1 -- PS-Simulink Converter4/LConn1
  Voltage/RConn1 -- PS-Simulink Converter5/LConn1

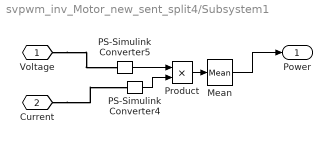
== system svpwm_inv_Motor_new_sent_split4/Subsystem1 ==
  Mean : spsMeanLib/Mean  Freq=5000  Vinit=0  Ts=0
  PS-Simulink Converter4 : nesl_utility/PS-Simulink Converter  PhysicalDomain=network_engine_domain  SubClassName=ps_output  LeftPortType=input  RightPortType=output  PseudoPeriodic=off  Frequencies=[]  VectorFormat=inherit  Unit=inherit  AffineConversion=off
  PS-Simulink Converter5 : nesl_utility/PS-Simulink Converter  PhysicalDomain=network_engine_domain  SubClassName=ps_output  LeftPortType=input  RightPortType=output  PseudoPeriodic=off  Frequencies=[]  VectorFormat=inherit  Unit=inherit  AffineConversion=off
  Product : Product
  Voltage : PMIOPort  Side=Left
  Current : PMIOPort  Port=2  Side=Left
  Power : Outport
  wires:
  Mean/1 -> Power/1
  PS-Simulink Converter4/1 -> Product/2
  PS-Simulink Converter5/1 -> Product/1
  Product/1 -> Mean/1
  connections:
  Voltage/RConn1 -- PS-Simulink Converter5/LConn1
  Current/RConn1 -- PS-Simulink Converter4/LConn1

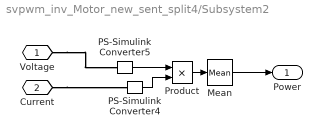
== system svpwm_inv_Motor_new_sent_split4/Subsystem2 ==
  Mean : spsMeanLib/Mean  Freq=5000  Vinit=0  Ts=0
  PS-Simulink Converter4 : nesl_utility/PS-Simulink Converter  PhysicalDomain=network_engine_domain  SubClassName=ps_output  LeftPortType=input  RightPortType=output  PseudoPeriodic=off  Frequencies=[]  VectorFormat=inherit  Unit=inherit  AffineConversion=off
  PS-Simulink Converter5 : nesl_utility/PS-Simulink Converter  PhysicalDomain=network_engine_domain  SubClassName=ps_output  LeftPortType=input  RightPortType=output  PseudoPeriodic=off  Frequencies=[]  VectorFormat=inherit  Unit=inherit  AffineConversion=off
  Product : Product
  Voltage : PMIOPort  Side=Left
  Current : PMIOPort  Port=2  Side=Left
  Power : Outport
  wires:
  Mean/1 -> Power/1
  PS-Simulink Converter4/1 -> Product/2
  PS-Simulink Converter5/1 -> Product/1
  Product/1 -> Mean/1
  connections:
  Voltage/RConn1 -- PS-Simulink Converter5/LConn1
  Current/RConn1 -- PS-Simulink Converter4/LConn1

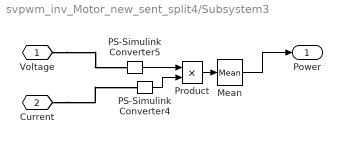
== system svpwm_inv_Motor_new_sent_split4/Subsystem3 ==
  Mean : spsMeanLib/Mean  Freq=5000  Vinit=0  Ts=0
  PS-Simulink Converter4 : nesl_utility/PS-Simulink Converter  PhysicalDomain=network_engine_domain  SubClassName=ps_output  LeftPortType=input  RightPortType=output  PseudoPeriodic=off  Frequencies=[]  VectorFormat=inherit  Unit=inherit  AffineConversion=off
  PS-Simulink Converter5 : nesl_utility/PS-Simulink Converter  PhysicalDomain=network_engine_domain  SubClassName=ps_output  LeftPortType=input  RightPortType=output  PseudoPeriodic=off  Frequencies=[]  VectorFormat=inherit  Unit=inherit  AffineConversion=off
  Product : Product
  Voltage : PMIOPort  Side=Left
  Current : PMIOPort  Port=2  Side=Left
  Power : Outport
  wires:
  Product/1 -> Mean/1
  PS-Simulink Converter5/1 -> Product/1
  PS-Simulink Converter4/1 -> Product/2
  Mean/1 -> Power/1
  connections:
  Current/RConn1 -- PS-Simulink Converter4/LConn1
  Voltage/RConn1 -- PS-Simulink Converter5/LConn1

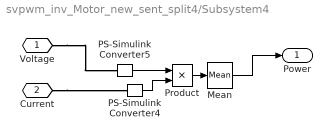
== system svpwm_inv_Motor_new_sent_split4/Subsystem4 ==
  Mean : spsMeanLib/Mean  Freq=5000  Vinit=0  Ts=0
  PS-Simulink Converter4 : nesl_utility/PS-Simulink Converter  PhysicalDomain=network_engine_domain  SubClassName=ps_output  LeftPortType=input  RightPortType=output  PseudoPeriodic=off  Frequencies=[]  VectorFormat=inherit  Unit=inherit  AffineConversion=off
  PS-Simulink Converter5 : nesl_utility/PS-Simulink Converter  PhysicalDomain=network_engine_domain  SubClassName=ps_output  LeftPortType=input  RightPortType=output  PseudoPeriodic=off  Frequencies=[]  VectorFormat=inherit  Unit=inherit  AffineConversion=off
  Product : Product
  Voltage : PMIOPort  Side=Left
  Current : PMIOPort  Port=2  Side=Left
  Power : Outport
  wires:
  Mean/1 -> Power/1
  PS-Simulink Converter4/1 -> Product/2
  PS-Simulink Converter5/1 -> Product/1
  Product/1 -> Mean/1
  connections:
  Voltage/RConn1 -- PS-Simulink Converter5/LConn1
  Current/RConn1 -- PS-Simulink Converter4/LConn1

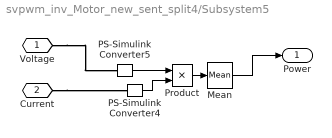
== system svpwm_inv_Motor_new_sent_split4/Subsystem5 ==
  Mean : spsMeanLib/Mean  Freq=5000  Vinit=0  Ts=0
  PS-Simulink Converter4 : nesl_utility/PS-Simulink Converter  PhysicalDomain=network_engine_domain  SubClassName=ps_output  LeftPortType=input  RightPortType=output  PseudoPeriodic=off  Frequencies=[]  VectorFormat=inherit  Unit=inherit  AffineConversion=off
  PS-Simulink Converter5 : nesl_utility/PS-Simulink Converter  PhysicalDomain=network_engine_domain  SubClassName=ps_output  LeftPortType=input  RightPortType=output  PseudoPeriodic=off  Frequencies=[]  VectorFormat=inherit  Unit=inherit  AffineConversion=off
  Product : Product
  Voltage : PMIOPort  Side=Left
  Current : PMIOPort  Port=2  Side=Left
  Power : Outport
  wires:
  Product/1 -> Mean/1
  PS-Simulink Converter5/1 -> Product/1
  PS-Simulink Converter4/1 -> Product/2
  Mean/1 -> Power/1
  connections:
  Current/RConn1 -- PS-Simulink Converter4/LConn1
  Voltage/RConn1 -- PS-Simulink Converter5/LConn1
